simulink model "BangBangAbs"  (R2026b)
undefined symbols (not defined in the file): CtrlBcuTrlrBrkGain, DiscIntNeverNeededParam
libraries: simulink x4, autolibutils x1
settings Model: Creator=The MathWorks, Inc.  LastModifiedBy=The MathWorks, Inc.

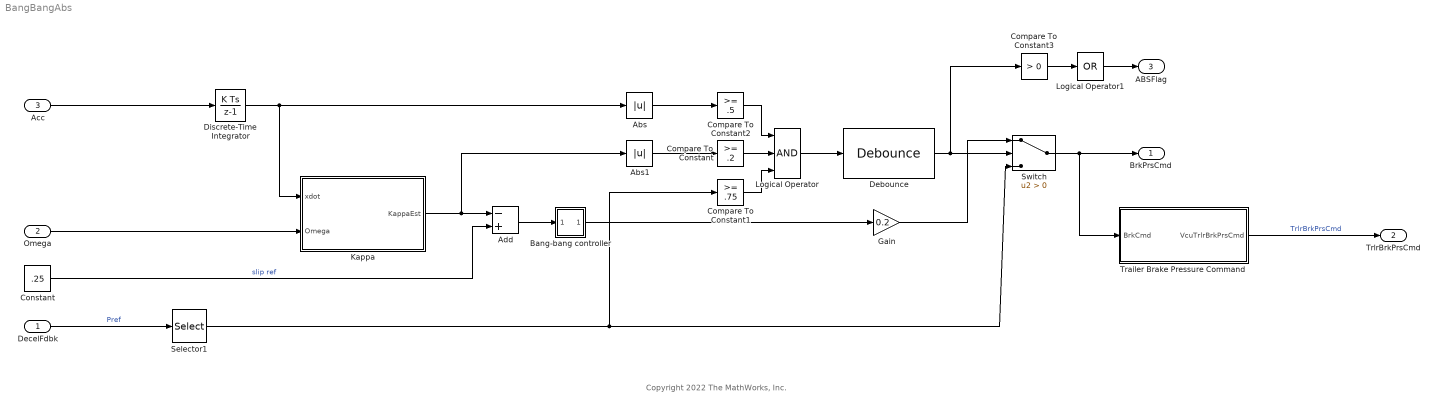
== system BangBangAbs ==
  note: Copyright 2022 The MathWorks, Inc.
  DecelFdbk : Inport  OutDataTypeStr=double  PortDimensions=1
  Omega : Inport  Port=2  OutDataTypeStr=double  PortDimensions=4
  Acc : Inport  Port=3  OutDataTypeStr=double  PortDimensions=1
  Abs : Abs  SaturateOnIntegerOverflow=off
  Abs1 : Abs  SaturateOnIntegerOverflow=off
  Add : Sum  Inputs=-+
  Bang-bang controller : Subsystem  mask(Sign){}
      mask help: y = sign(x)
      mask Help: Sign Function:\n\t\t\ty = 1 if x > 0\n\t\t\ty = 0 if x = 0\n\t\t\ty = -1 if x < 0
      mask Display: plot(-50,-50,50,50,[-50,50],[0,0],[0,0],[-50,50],[-40,0],[-30,-30],[0,40],[30,30])
  Compare To Constant : simulink/Logic and Bit Operations/Compare To Constant  relop=>=  const=.2  OutDataTypeStr=boolean
  Compare To Constant1 : simulink/Logic and Bit Operations/Compare To Constant  relop=>=  const=.75  OutDataTypeStr=boolean
  Compare To Constant2 : simulink/Logic and Bit Operations/Compare To Constant  relop=>=  const=.5  OutDataTypeStr=boolean
  Compare To Constant3 : simulink/Logic and Bit Operations/Compare To Constant  relop=>  const=0  OutDataTypeStr=boolean  ZeroCross=off
  Constant : Constant  Value=.25
  Debounce : autolibutils/Debounce  DbcOn_Cnts=.1*.001  DbcOff_Cnts=.1*.001  aMode=2
  Discrete-Time Integrator : DiscreteIntegrator  SampleTime=-1  LimitOutput=on  LowerSaturationLimit=0  ICPrevOutput=DiscIntNeverNeededParam  ICPrevScaledInput=DiscIntNeverNeededParam
  Gain : Gain  Gain=0.2
  Kappa : Subsystem  TreatAsAtomicUnit=on
  Logical Operator : Logic  Inputs=3  AllPortsSameDT=off  OutDataTypeStr=boolean
  Logical Operator1 : Logic  Operator=OR  Inputs=1  AllPortsSameDT=off  OutDataTypeStr=boolean
  Selector1 : Selector  InputPortWidth=1  IndexOptions=Index vector (dialog)  Indices=[1 1 1 1]  OutputSizes=1  RuntimeRangeChecks=off
  Switch : Switch  Criteria=u2 > Threshold  ZeroCross=off  SaturateOnIntegerOverflow=off  InputSameDT=off
  Trailer Brake Pressure Command : Subsystem
  BrkPrsCmd : Outport  OutDataTypeStr=double  PortDimensions=4  VectorParamsAs1DForOutWhenUnconnected=off
  TrlrBrkPrsCmd : Outport  Port=2  PortDimensions=6  VectorParamsAs1DForOutWhenUnconnected=off
  ABSFlag : Outport  Port=3
  wires:
  Selector1/1 -> Compare To Constant1/1, Switch/3
  Gain/1 -> Switch/1
  Compare To Constant3/1 -> Logical Operator1/1
  Kappa/1(KappaEst) -> Add/1, Abs1/1
  Compare To Constant/1 -> Logical Operator/2
  Compare To Constant1/1 -> Logical Operator/3
  Compare To Constant2/1 -> Logical Operator/1
  Debounce/1 -> Compare To Constant3/1, Switch/2
  Logical Operator/1 -> Debounce/1
  Add/1 -> Bang-bang controller/1(in_1)
  Acc/1 -> Discrete-Time Integrator/1
  Discrete-Time Integrator/1 -> Kappa/1(xdot), Abs/1
  Constant/1 -> Add/2  "slip ref"
  DecelFdbk/1 -> Selector1/1  "Pref"
  Bang-bang controller/1(out_1) -> Gain/1
  Abs/1 -> Compare To Constant2/1
  Omega/1 -> Kappa/2(Omega)
  Switch/1 -> Trailer Brake Pressure Command/1(BrkCmd), BrkPrsCmd/1
  Trailer Brake Pressure Command/1(VcuTrlrBrkPrsCmd) -> TrlrBrkPrsCmd/1  "TrlrBrkPrsCmd"
  Abs1/1 -> Compare To Constant/1
  Logical Operator1/1 -> ABSFlag/1

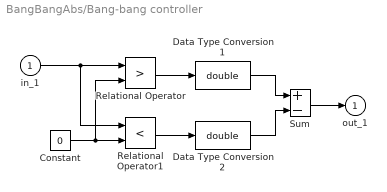
== system BangBangAbs/Bang-bang controller ==
  in_1 : Inport
  Constant : Constant  Value=0
  Data Type Conversion1 : DataTypeConversion  OutDataTypeStr=double
  Data Type Conversion2 : DataTypeConversion  OutDataTypeStr=double
  Relational Operator : RelationalOperator  Operator=>  OutDataTypeStr=boolean
  Relational Operator1 : RelationalOperator  Operator=<  OutDataTypeStr=boolean
  Sum : Sum  Inputs=+-  InputSameDT=on  SaturateOnIntegerOverflow=on  OutDataTypeStr=Inherit: Same as first input
  out_1 : Outport  InitialOutput=0  VectorParamsAs1DForOutWhenUnconnected=off
  wires:
  Data Type Conversion2/1 -> Sum/2
  Data Type Conversion1/1 -> Sum/1
  Sum/1 -> out_1/1
  Relational Operator/1 -> Data Type Conversion1/1
  Relational Operator1/1 -> Data Type Conversion2/1
  Constant/1 -> Relational Operator/2, Relational Operator1/2
  in_1/1 -> Relational Operator1/1, Relational Operator/1

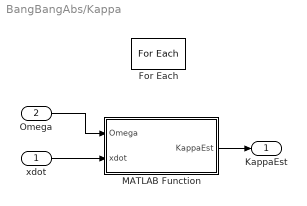
== system BangBangAbs/Kappa ==
  xdot : Inport
  Omega : Inport  Port=2  Partition=on  PartitionDimension=1  PartitionWidth=1  PartitionOffset=0
  For Each : ForEach  DisableCoverage=on
  MATLAB Function : MATLAB Function  TreatAsAtomicUnit=on
  KappaEst : Outport  ConcatenationDimension=1
  wires:
  MATLAB Function/1(KappaEst) -> KappaEst/1
  xdot/1 -> MATLAB Function/2(xdot)
  Omega/1 -> MATLAB Function/1(Omega)

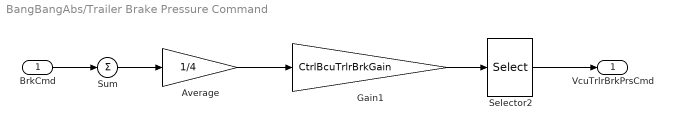
== system BangBangAbs/Trailer Brake Pressure Command ==
  BrkCmd : Inport
  Average : Gain  Gain=1/4
  Gain1 : Gain  Gain=CtrlBcuTrlrBrkGain
  Selector2 : Selector  InputPortWidth=1  IndexOptions=Index vector (dialog)  Indices=[1 1 1 1 1 1]  OutputSizes=1  RuntimeRangeChecks=off
  Sum : Sum  Inputs=+
  VcuTrlrBrkPrsCmd : Outport
  wires:
  Gain1/1 -> Selector2/1
  Average/1 -> Gain1/1
  BrkCmd/1 -> Sum/1
  Sum/1 -> Average/1
  Selector2/1 -> VcuTrlrBrkPrsCmd/1

== matlab function BangBangAbs/Kappa/MATLAB Function ==
  data: Omega input; xdot input; KappaEst output
function KappaEst = fcn(Omega, xdot)

Re = 0.29;
KappaEst = 0;
WhlSpd = Omega * Re;

if xdot*WhlSpd ~= 0
    KappaEst = (WhlSpd - xdot)/max([abs(xdot) abs(WhlSpd)]);
end
